simulink model "Diff_Simulink_SimscapeModel"  (R2022b)
settings: Solver=daessc  StartTime=0.0  StopTime=0.03  RelTol=1e-3
undefined symbols (not defined in the file): Duty, Ro, Vin
settings Model: Creator=ykamatan  LastModifiedBy=ykamatan

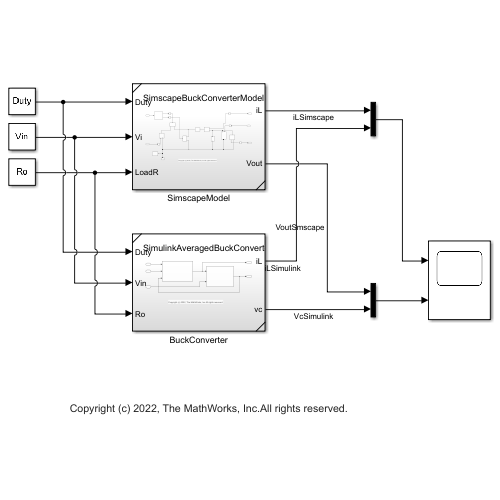
[thumbnail: Simulink's stored preview of the top-level diagram]
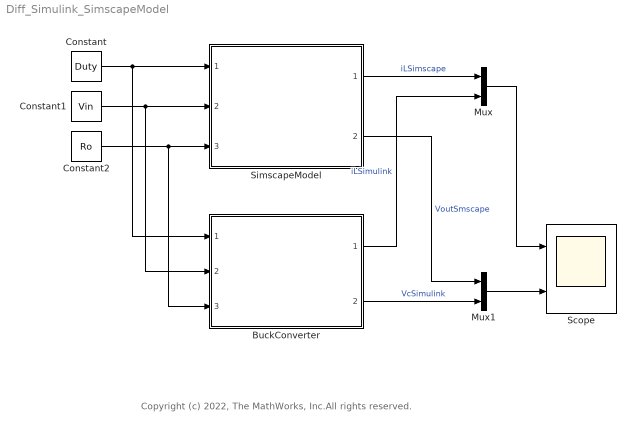
== system Diff_Simulink_SimscapeModel ==
  note: Copyright (c) 2022, The MathWorks, Inc.All rights reserved.
  BuckConverter : Subsystem  ReferencedSubsystem=SimulinkAveragedBuckConverterModel
  Constant : Constant  Value=Duty
  Constant1 : Constant  Value=Vin
  Constant2 : Constant  Value=Ro
  Mux : Mux  Inputs=2
  Mux1 : Mux  Inputs=2
  Scope : Scope  NumInputPorts=2
  SimscapeModel : Subsystem  ReferencedSubsystem=SimscapeBuckConverterModel
  wires:
  Constant2/1 -> BuckConverter/3, SimscapeModel/3
  Constant/1 -> BuckConverter/1, SimscapeModel/1
  Constant1/1 -> BuckConverter/2, SimscapeModel/2
  SimscapeModel/1 -> Mux/1  "iLSimscape"
  BuckConverter/1 -> Mux/2  "iLSimulink"
  BuckConverter/2 -> Mux1/2  "VcSimulink"
  SimscapeModel/2 -> Mux1/1  "VoutSmscape"
  Mux1/1 -> Scope/2
  Mux/1 -> Scope/1
